simulink model "TST_DReqSwt_DD"  (R2016b)
settings: Solver=FixedStepDiscrete  StartTime=0.0  StopTime=simTime  FixedStep=sampleTime  RelTol=1e-3
libraries: simulink x1
settings Model: Creator=zhoudefeng  LastModifiedBy=zhoudefeng
settings DebuggingCC: SignalRangeChecking=error

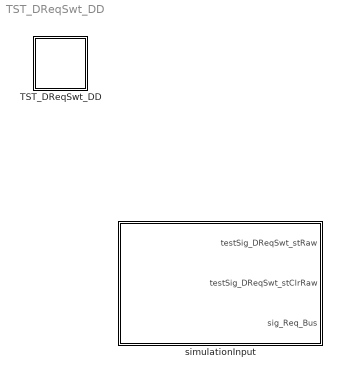
== system TST_DReqSwt_DD ==
  TST_DReqSwt_DD : Subsystem
  simulationInput : Subsystem

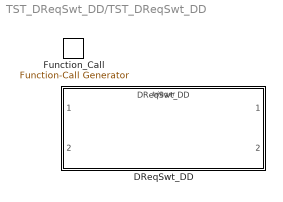
== system TST_DReqSwt_DD/TST_DReqSwt_DD ==
  DReqSwt_DD : ModelReference  ModelNameDialog=DReqSwt_DD  SimulationMode=Normal  ModelReferenceVersion=1.10  TriggerPortName=function  TriggerPortTriggerType=function-call  TriggerPortStatesWhenEnabling=held
  Function_Call : simulink/Ports & Subsystems/Function-Call Generator  sample_time=sampleTime  numberOfIterations=1

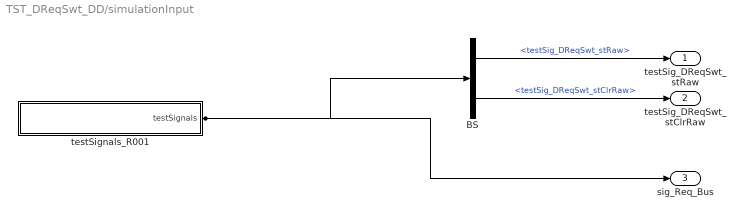
== system TST_DReqSwt_DD/simulationInput ==
  BS : BusSelector  OutputSignals=testSig_DReqSwt_stRaw,testSig_DReqSwt_stClrRaw
  testSignals_R001 : Subsystem
  testSig_DReqSwt_stRaw : Outport
  testSig_DReqSwt_stClrRaw : Outport  Port=2
  sig_Req_Bus : Outport  Port=3
  wires:
  BS/1 -> testSig_DReqSwt_stRaw/1  "<testSig_DReqSwt_stRaw>"
  BS/2 -> testSig_DReqSwt_stClrRaw/1  "<testSig_DReqSwt_stClrRaw>"
  testSignals_R001/1(testSignals) -> BS/1, sig_Req_Bus/1

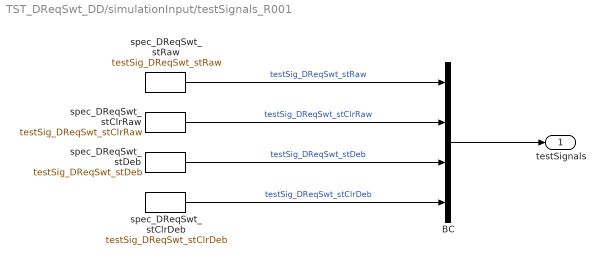
== system TST_DReqSwt_DD/simulationInput/testSignals_R001 ==
  BC : BusCreator  Inputs=4
  spec_DReqSwt_stClrDeb : FromWorkspace  VariableName=testSig_DReqSwt_stClrDeb  Interpolate=off  OutputAfterFinalValue=Holding final value
  spec_DReqSwt_stClrRaw : FromWorkspace  VariableName=testSig_DReqSwt_stClrRaw  Interpolate=off  OutputAfterFinalValue=Holding final value
  spec_DReqSwt_stDeb : FromWorkspace  VariableName=testSig_DReqSwt_stDeb  Interpolate=off  OutputAfterFinalValue=Holding final value
  spec_DReqSwt_stRaw : FromWorkspace  VariableName=testSig_DReqSwt_stRaw  Interpolate=off  OutputAfterFinalValue=Holding final value
  testSignals : Outport
  wires:
  BC/1 -> testSignals/1
  spec_DReqSwt_stRaw/1 -> BC/1  "testSig_DReqSwt_stRaw"
  spec_DReqSwt_stClrRaw/1 -> BC/2  "testSig_DReqSwt_stClrRaw"
  spec_DReqSwt_stDeb/1 -> BC/3  "testSig_DReqSwt_stDeb"
  spec_DReqSwt_stClrDeb/1 -> BC/4  "testSig_DReqSwt_stClrDeb"
